simulink model "Ranging_Estimator0"  (R2020b)
settings: Solver=FixedStepDiscrete  StartTime=0.0  StopTime=inf  FixedStep=0.000001  RelTol=1e-3  EnableMultiTasking=on
settings Model: SILPILModeSetting=veronly  ExtModeTrigDuration=2  Creator=GUO HUI  LastModifiedBy=GUO HUI
settings DataIOCC: SaveOutput=off  SaveTime=off
settings OptimizationCC: EnhancedBackFolding=on  PassReuseOutputArgsAs=Individual arguments  MaxStackSize=64  OptimizeBlockOrder=speed  DifferentSizesBufferReuse=on  OptimizationCustomize=off  EfficientTunableParamExpr=on
settings DebuggingCC: ParameterTunabilityLossMsg=error
settings HardwareCC: ProdBitPerInt=16  ProdBitPerPointer=16  ProdBitPerSizeT=16  ProdBitPerPtrDiffT=16  ProdLargestAtomicFloat=None  ProdWordSize=8  ProdHWDeviceType=Atmel->AVR
settings SFSimCC: MATLABDynamicMemAlloc=off
settings RTWCC: Description=Embedded Coder  SystemTargetFile=ert.tlc  HardwareBoard=Arduino Uno  GenCodeOnly=on  TemplateMakefile=ert_default_tmf  GenerateReport=on  Toolchain=Arduino AVR  BuildConfiguration=Faster Runs  IncludeHyperlinkInReport=on  LaunchReport=on  GenerateTraceInfo=on  GenerateCodeMetricsReport=on
settings CodeAppCC: ForceParamTrailComments=on  IgnoreCustomStorageClasses=off  OperatorAnnotations=on  SimulinkDataObjDesc=on  SFDataObjDesc=on  InsertBlockDesc=on
settings ERTTargetCC: CodeInterfacePackaging=Reusable function  SupportContinuousTime=on  SupportVariableSizeSignals=on  ExtModeStaticAllocSize=250  ERTFilePackagingFormat=Compact
settings ConfigComp: CovEnable=on  CovScope=Subsystem  RecordCoverage=on  CovSaveSingleToWorkspaceVar=on  CovExternalEMLEnable=off  CovSFcnEnable=off

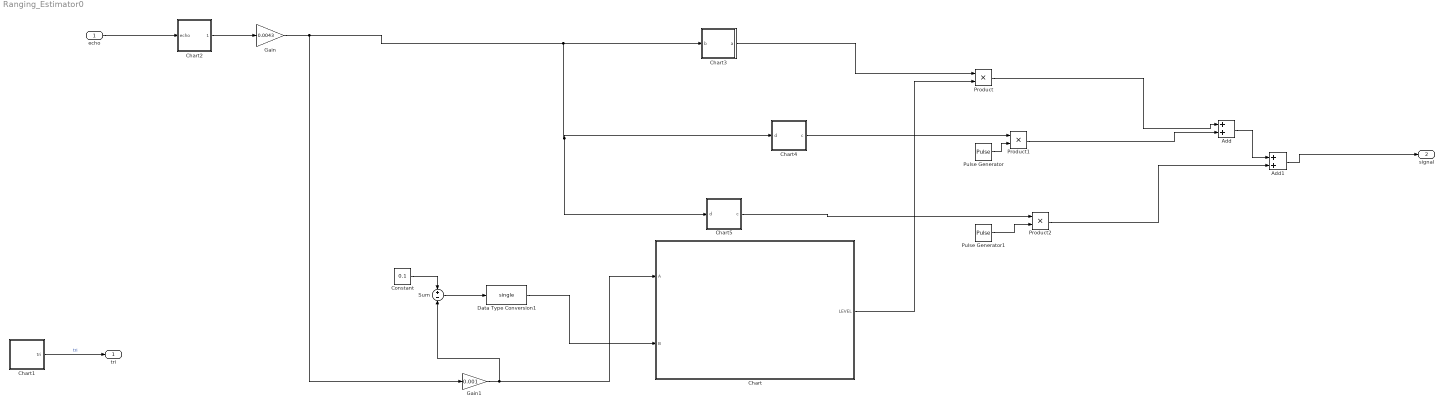
== system Ranging_Estimator0 ==
  echo : Inport  OutDataTypeStr=double  PortDimensions=1
  Add : Sum
  Add1 : Sum
  Chart : Stateflow chart  TreatAsAtomicUnit=on
  Chart1 : Stateflow chart  TreatAsAtomicUnit=on
  Chart2 : Stateflow chart  TreatAsAtomicUnit=on
  Chart3 : Stateflow chart  TreatAsAtomicUnit=on
  Chart4 : Stateflow chart  TreatAsAtomicUnit=on
  Chart5 : Stateflow chart  TreatAsAtomicUnit=on
  Constant : Constant  Value=0.1
  Data Type Conversion1 : DataTypeConversion  OutDataTypeStr=single
  Gain : Gain  Gain=0.0043
  Gain1 : Gain  Gain=0.001
  Product : Product
  Product1 : Product
  Product2 : Product
  Pulse Generator : DiscretePulseGenerator  PulseType=Time based  Period=0.5  PulseWidth=50
  Pulse Generator1 : DiscretePulseGenerator  PulseType=Time based  Period=1  PulseWidth=50
  Sum : Sum  Inputs=+-
  tri : Outport  OutDataTypeStr=double  PortDimensions=1  SampleTime=[9.9999999999999995e-07,0]
  signal : Outport  Port=2  OutDataTypeStr=double  PortDimensions=1  SampleTime=[9.9999999999999995e-07,0]
  wires:
  Chart2/1(echodis) -> Gain/1
  Chart3/1(a) -> Product/1
  echo/1 -> Chart2/1(echo)
  Chart1/1(tri) -> tri/1  "tri"
  Pulse Generator/1 -> Product1/2
  Product1/1 -> Add/2
  Product/1 -> Add/1
  Product2/1 -> Add1/2
  Add/1 -> Add1/1
  Pulse Generator1/1 -> Product2/2
  Chart5/1(c) -> Product2/1
  Sum/1 -> Data Type Conversion1/1
  Data Type Conversion1/1 -> Chart/2(B)
  Constant/1 -> Sum/1
  Gain1/1 -> Chart/1(A), Sum/2
  Chart/1(LEVEL) -> Product/2
  Chart4/1(c) -> Product1/1
  Add1/1 -> signal/1
  Gain/1 -> Gain1/1, Chart5/1(d), Chart4/1(d), Chart3/1(b)

== stateflow chart Ranging_Estimator0/Chart ==
  state START
    en:LEVEL=1
  state OFF
    en:LEVEL=0
  (default) -> START
  START -> OFF : [after(A,sec)]
  OFF -> START : [after(B,sec)]
  data: A input; B input; LEVEL output

== stateflow chart Ranging_Estimator0/Chart2 ==
  state start
    en:loop=0;
    counter=5;
  state count
    du:counter=counter+1;
    ex:echodis=counter
  state wait
  state exit
  (default) -> start
  count -> wait : [echo==0]{loop=loop+1}
  start -> wait
  wait -> exit [order 2] : [loop>3]
  wait -> count [order 1] : [echo==1]
  data: echo input; counter local; echodis output; loop local

== stateflow chart Ranging_Estimator0/Chart4 ==
  state wait
  state output
    en:c=1;
  (default) -> wait
  wait -> output : [d<10&&d>0||d>100]
  data: d input; c output

== stateflow chart Ranging_Estimator0/Chart5 ==
  state input
  state wait
  state output
    en:c=1;
  (default) -> input
  wait -> output : [d==0]
  input -> wait : after(0.07,sec)
  data: d input; c output

== stateflow chart Ranging_Estimator0/Chart3 ==
  state wait1
  state out
    en:a=1;
  (default) -> wait1
  wait1 -> out : [b>=10&&b<100]
  data: a output; b input

== stateflow chart Ranging_Estimator0/Chart1 ==
  state state_on1
    en:tri=1;
  state state_off
    en:tri=0;
  (default) -> state_on1
  state_on1 -> state_off : after(10,usec)
  state_off -> state_on1 : after(60,msec)
  data: tri output
